simulink model "vehicle_psd"  (R2017a)
settings: Solver=VariableStepAuto  StartTime=0.0  StopTime=200  RelTol=1e-3
InitFcn:
  | if ~exist('Ts')
  |     Ts = 1;
  | end
libraries: elvio x16, simulink x4
settings Model: Creator=tstef  LastModifiedBy=thomas

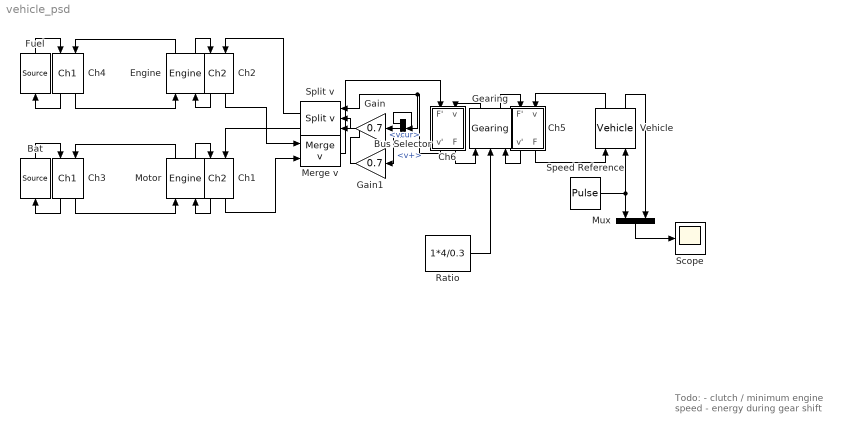
== system vehicle_psd ==
  note: Todo:
      | - clutch / minimum engine speed
      | - energy during gear shift
  Bat : elvio/Basics/Source
  Bus Selector : BusSelector  OutputSignals=vcur,v+
  Ch1 : elvio/Basics/Ch2
  Ch2 : elvio/Basics/Ch2
  Ch3 : elvio/Basics/Ch1
  Ch4 : elvio/Basics/Ch1
  Ch5 : Subsystem
  Ch6 : Subsystem
  Engine : elvio/Drive/Engine  Tmax=[40 50 60 80 100 120 150 200 300 500]  Tmin=0  Tfrict=10  Ploss=1000  eff=0
  Fuel : elvio/Basics/Source
  Gain : Gain  Gain=0.7
  Gain1 : Gain  Gain=0.7
  Gearing : elvio/Basics/Gearing
  Merge v : elvio/Basics/Merge v
  Motor : elvio/Drive/Engine  Tmax=[40 50 60 80 100 120 150 200 300 500]  Tmin=0  Tfrict=10  Ploss=1000  eff=0
  Mux : Mux  Inputs=2
  Ratio : Constant  Value=1*4/0.3
  Scope : Scope
  Speed Reference : DiscretePulseGenerator  PulseType=Time based  Amplitude=20  Period=100  PulseWidth=49.9
  Split v : elvio/Basics/Split v
  Vehicle : elvio/Drive/Vehicle  m=1200  Froll=15  Aeff=0.4  Tbrake=5000  n=[10 1]
  wires:
  Ratio/1 -> Gearing/2
  Mux/1 -> Scope/1
  Fuel/1 -> Ch4/1
  Ch4/1 -> Fuel/1
  Ch2/1 -> Engine/2
  Ch4/2 -> Engine/1
  Engine/1 -> Ch4/2
  Engine/2 -> Ch2/1
  Motor/2 -> Ch1/1
  Motor/1 -> Ch3/2
  Ch3/2 -> Motor/1
  Ch1/1 -> Motor/2
  Ch3/1 -> Bat/1
  Bat/1 -> Ch3/1
  Split v/1 -> Ch2/2
  Split v/2 -> Ch1/2
  Ch2/2 -> Merge v/1
  Ch1/2 -> Merge v/2
  Merge v/1 -> Ch6/1(F')
  Gearing/2 -> Ch5/1(F')
  Ch5/1(v') -> Gearing/3
  Ch5/2(F) -> Vehicle/1
  Vehicle/2 -> Mux/2
  Vehicle/1 -> Ch5/2(v)
  Speed Reference/1 -> Vehicle/2, Mux/1
  Ch6/1(v') -> Bus Selector/1, Split v/1
  Gain/1 -> Split v/2
  Bus Selector/1 -> Gain/1  "<vcur>"
  Gearing/1 -> Ch6/2(v)
  Ch6/2(F) -> Gearing/1
  Gain1/1 -> Split v/3
  Bus Selector/2 -> Gain1/1  "<v+>"

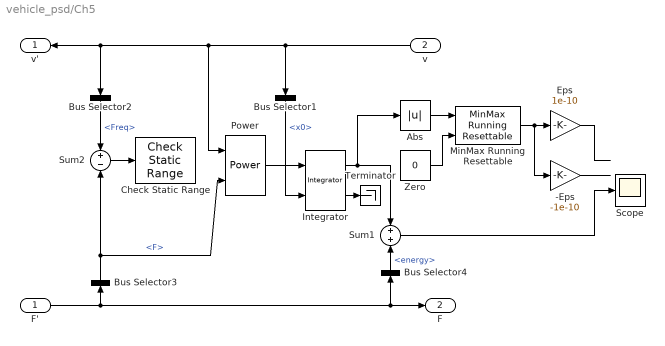
== system vehicle_psd/Ch5 ==
  F' : Inport
  v : Inport  Port=2
  -Eps : Gain  Gain=-1e-10
  Abs : Abs  ZeroCross=off
  Bus Selector1 : BusSelector  OutputSignals=info.x0
  Bus Selector2 : BusSelector  OutputSignals=Freq
  Bus Selector3 : BusSelector  OutputSignals=F
  Bus Selector4 : BusSelector  OutputSignals=energy
  Check Static Range : simulink/Model Verification/Check  Static Range  Description=-1e-10 <= u <= 1e-10  max=1e-10  max_included=on  min=-1e-10  min_included=on  enabled=on  stopWhenAssertionFail=on  export=off  icon=graphic
      settings: SourceProductName=Simulink  SourceProductBaseCode=SL
  Eps : Gain  Gain=1e-10
  Integrator : elvio/Utilities/Integrator  Ts=Ts
  MinMax Running Resettable : simulink/Math Operations/MinMax Running Resettable  Function=max  vinit=1e-6
  Power : elvio/Basics/Power
  Scope : Scope
  Sum1 : Sum
  Sum2 : Sum  Inputs=+-
  Terminator : Terminator
  Zero : Constant  Value=0
  v' : Outport
  F : Outport  Port=2
  wires:
  Sum2/1 -> Check Static Range/1
  Bus Selector2/1 -> Sum2/1  "<Freq>"
  Zero/1 -> MinMax Running Resettable/2
  Integrator/1 -> Abs/1, Sum1/1
  Integrator/2 -> Terminator/1
  v/1 -> v'/1, Bus Selector2/1, Power/1, Bus Selector1/1
  Bus Selector1/1 -> Integrator/2  "<x0>"
  F'/1 -> Bus Selector3/1, Bus Selector4/1, F/1
  Bus Selector4/1 -> Sum1/2  "<energy>"
  Sum1/1 -> Scope/1
  Power/1 -> Integrator/1
  Abs/1 -> MinMax Running Resettable/1
  Eps/1 -> ?
  MinMax Running Resettable/1 -> Eps/1, -Eps/1
  -Eps/1 -> ?
  Bus Selector3/1 -> Sum2/2, Power/2  "<F>"

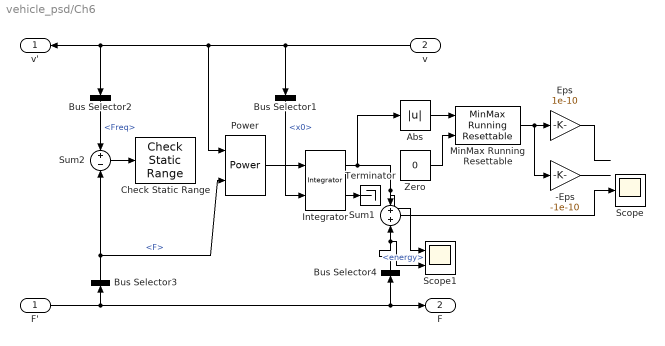
== system vehicle_psd/Ch6 ==
  F' : Inport
  v : Inport  Port=2
  -Eps : Gain  Gain=-1e-10
  Abs : Abs  ZeroCross=off
  Bus Selector1 : BusSelector  OutputSignals=info.x0
  Bus Selector2 : BusSelector  OutputSignals=Freq
  Bus Selector3 : BusSelector  OutputSignals=F
  Bus Selector4 : BusSelector  OutputSignals=energy
  Check Static Range : simulink/Model Verification/Check  Static Range  Description=-1e-10 <= u <= 1e-10  max=1e-10  max_included=on  min=-1e-10  min_included=on  enabled=on  stopWhenAssertionFail=on  export=off  icon=graphic
      settings: SourceProductName=Simulink  SourceProductBaseCode=SL
  Eps : Gain  Gain=1e-10
  Integrator : elvio/Utilities/Integrator  Ts=Ts
  MinMax Running Resettable : simulink/Math Operations/MinMax Running Resettable  Function=max  vinit=1e-6
  Power : elvio/Basics/Power
  Scope : Scope
  Scope1 : Scope  NumInputPorts=2
  Sum1 : Sum
  Sum2 : Sum  Inputs=+-
  Terminator : Terminator
  Zero : Constant  Value=0
  v' : Outport
  F : Outport  Port=2
  wires:
  Bus Selector3/1 -> Power/2, Sum2/2  "<F>"
  -Eps/1 -> ?
  MinMax Running Resettable/1 -> -Eps/1, Eps/1
  Eps/1 -> ?
  Abs/1 -> MinMax Running Resettable/1
  Power/1 -> Integrator/1
  Sum1/1 -> Scope/1
  Bus Selector4/1 -> Scope1/2, Sum1/2  "<energy>"
  F'/1 -> F/1, Bus Selector4/1, Bus Selector3/1
  Bus Selector1/1 -> Integrator/2  "<x0>"
  v/1 -> Bus Selector1/1, Power/1, Bus Selector2/1, v'/1
  Integrator/2 -> Terminator/1
  Integrator/1 -> Scope1/1, Sum1/1, Abs/1
  Zero/1 -> MinMax Running Resettable/2
  Bus Selector2/1 -> Sum2/1  "<Freq>"
  Sum2/1 -> Check Static Range/1
